simulink library "ada"  (Simulink 8.1)
settings: Solver=ode1  StartTime=0.0  StopTime=Inf  FixedStep=0.001  RelTol=1e-3
PostLoadFcn:
  | , if any(exist('dsrtsu_mdlpostloadfcn', 'file') == [2, 3, 6]), try dsrtsu_mdlpostloadfcn('Execute', bdroot); catch fprintf('Error in PostLoadFcn (dsrtsu_mdlpostloadfcn) for model "%s":\n %s\n', bdroot, lasterr); end, end,
settings Model: DSRTSU_INTERNAL_RTI_VER=450  DSRTSU_INTERNAL_RTI_TYPE=rti1401  RTICANMMDATA=struct('GeneralSetupData',struct('modelroot','D:\ELN150201\Phase3\trunk\Application\AdasDragon\software\sw_development\arch\app\ada','generalsettings',struct('filesettings',struct('destfolder',struct('Name','RTICANMM_FILES','Check',1),'buildfolder',struct('Name','.','Check',1),'AbsDestfolder',struct('Name','D:\ELN150201\Phase3\trunk\Application\AdasDragon\software\sw_development\arch\app\ada\RTICANMM_FILES'),'AbsBuildfolder',struct('Name','D:\ELN150201\Phase3\trunk\Application\AdasDragon\software\sw_development\arch\app\ada'))),'options',struct('addpaths',1,'rmpaths',1,'addtrcexclusion',logical(1),'cannavigator',struct('checkmonitoring',0),'show_usrtrc',0,'use_usrtrc',0),'advanced',struct('options',[1 1 1 1 1 1 1 1 1 1 1 1 1 1 1 1 1 1 1 1 1 1 1 1 1 1 1 1 1 1 1 1 1 1 1 1 1 1 1 1 1 1 1 1 1 1 1 1 1 1 1 1 1 1 1 1 1 1 1 1 1 1 1 1 1 1 1 1 1 1 1 1 1 1 1 1 1 1 1 1 1 1 1 1 1 1 1 1 1 1 1 1 1 1 1 1 1 1 1 1]),'MPSetup',{{}},'modelname','ada','block','ada'))  DSRTSU_INTERNAL_RTIFPGA=40  Creator=tescamilla  LastModifiedBy=AT015555

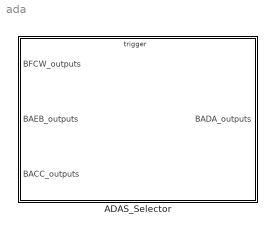
== system ada ==
  ADAS_Selector : Subsystem

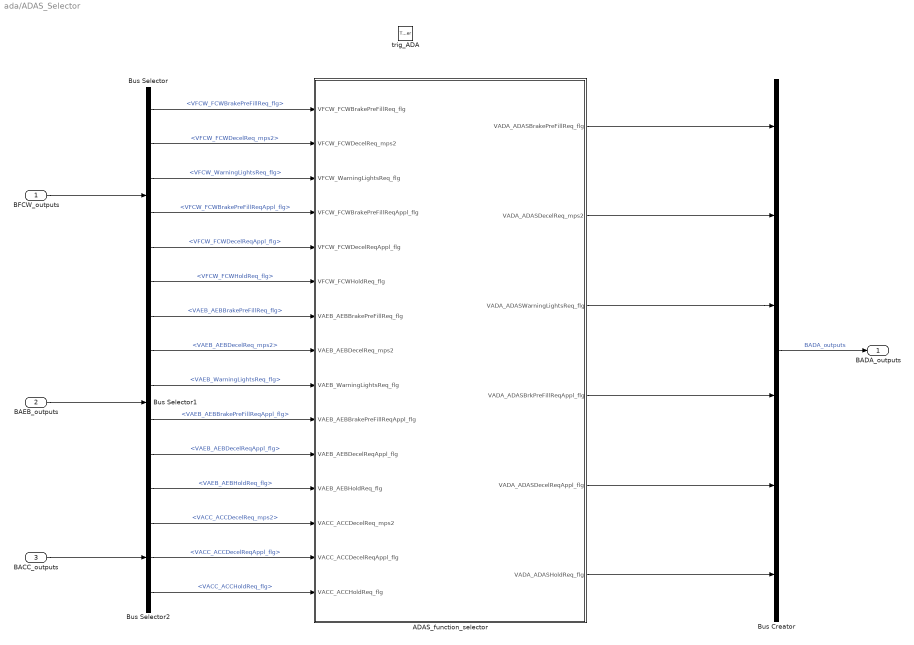
== system ada/ADAS_Selector ==
  BFCW_outputs : Inport  OutDataTypeStr=Bus: BFCW_outputs
  BAEB_outputs : Inport  Port=2  OutDataTypeStr=Bus: BAEB_outputs
  BACC_outputs : Inport  Port=3  OutDataTypeStr=Bus: BACC_outputs
  trig_ADA : TriggerPort  TriggerType=function-call
      settings: AttributesFormatString=State = %<StatesWhenEnabling>
  ADAS_function_selector : Subsystem
  Bus Creator : BusCreator  Inputs=6  OutDataTypeStr=Bus: BADA_outputs
  Bus Selector : BusSelector  OutputSignals=VFCW_FCWBrakePreFillReq_flg,VFCW_FCWDecelReq_mps2,VFCW_WarningLightsReq_flg,VFCW_FCWBrakePreFillReqAppl_flg,VFCW_FCWDecelReqAppl_flg,VFCW_FCWHoldReq_flg
  Bus Selector1 : BusSelector  OutputSignals=VAEB_AEBBrakePreFillReq_flg,VAEB_AEBDecelReq_mps2,VAEB_WarningLightsReq_flg,VAEB_AEBBrakePreFillReqAppl_flg,VAEB_AEBDecelReqAppl_flg,VAEB_AEBHoldReq_flg
  Bus Selector2 : BusSelector  OutputSignals=VACC_ACCDecelReq_mps2,VACC_ACCDecelReqAppl_flg,VACC_ACCHoldReq_flg
  BADA_outputs : Outport  OutDataTypeStr=Bus: BADA_outputs  LockScale=on
  wires:
  BFCW_outputs/1 -> Bus Selector/1
  BAEB_outputs/1 -> Bus Selector1/1
  Bus Selector1/5 -> ADAS_function_selector/11(VAEB_AEBDecelReqAppl_flg)  "<VAEB_AEBDecelReqAppl_flg>"
  Bus Selector1/1 -> ADAS_function_selector/7(VAEB_AEBBrakePreFillReq_flg)  "<VAEB_AEBBrakePreFillReq_flg>"
  Bus Selector/3 -> ADAS_function_selector/3(VFCW_WarningLightsReq_flg)  "<VFCW_WarningLightsReq_flg>"
  Bus Selector/6 -> ADAS_function_selector/6(VFCW_FCWHoldReq_flg)  "<VFCW_FCWHoldReq_flg>"
  Bus Selector/2 -> ADAS_function_selector/2(VFCW_FCWDecelReq_mps2)  "<VFCW_FCWDecelReq_mps2>"
  Bus Selector/5 -> ADAS_function_selector/5(VFCW_FCWDecelReqAppl_flg)  "<VFCW_FCWDecelReqAppl_flg>"
  Bus Selector/1 -> ADAS_function_selector/1(VFCW_FCWBrakePreFillReq_flg)  "<VFCW_FCWBrakePreFillReq_flg>"
  Bus Selector/4 -> ADAS_function_selector/4(VFCW_FCWBrakePreFillReqAppl_flg)  "<VFCW_FCWBrakePreFillReqAppl_flg>"
  Bus Selector1/3 -> ADAS_function_selector/9(VAEB_WarningLightsReq_flg)  "<VAEB_WarningLightsReq_flg>"
  Bus Selector1/2 -> ADAS_function_selector/8(VAEB_AEBDecelReq_mps2)  "<VAEB_AEBDecelReq_mps2>"
  Bus Selector1/4 -> ADAS_function_selector/10(VAEB_AEBBrakePreFillReqAppl_flg)  "<VAEB_AEBBrakePreFillReqAppl_flg>"
  Bus Selector1/6 -> ADAS_function_selector/12(VAEB_AEBHoldReq_flg)  "<VAEB_AEBHoldReq_flg>"
  ADAS_function_selector/1(VADA_ADASBrakePreFillReq_flg) -> Bus Creator/1
  Bus Creator/1 -> BADA_outputs/1  "BADA_outputs"
  ADAS_function_selector/3(VADA_ADASWarningLightsReq_flg) -> Bus Creator/3
  ADAS_function_selector/6(VADA_ADASHoldReq_flg) -> Bus Creator/6
  ADAS_function_selector/2(VADA_ADASDecelReq_mps2) -> Bus Creator/2
  ADAS_function_selector/5(VADA_ADASDecelReqAppl_flg) -> Bus Creator/5
  ADAS_function_selector/4(VADA_ADASBrkPreFillReqAppl_flg) -> Bus Creator/4
  BACC_outputs/1 -> Bus Selector2/1
  Bus Selector2/1 -> ADAS_function_selector/13(VACC_ACCDecelReq_mps2)  "<VACC_ACCDecelReq_mps2>"
  Bus Selector2/3 -> ADAS_function_selector/15(VACC_ACCHoldReq_flg)  "<VACC_ACCHoldReq_flg>"
  Bus Selector2/2 -> ADAS_function_selector/14(VACC_ACCDecelReqAppl_flg)  "<VACC_ACCDecelReqAppl_flg>"

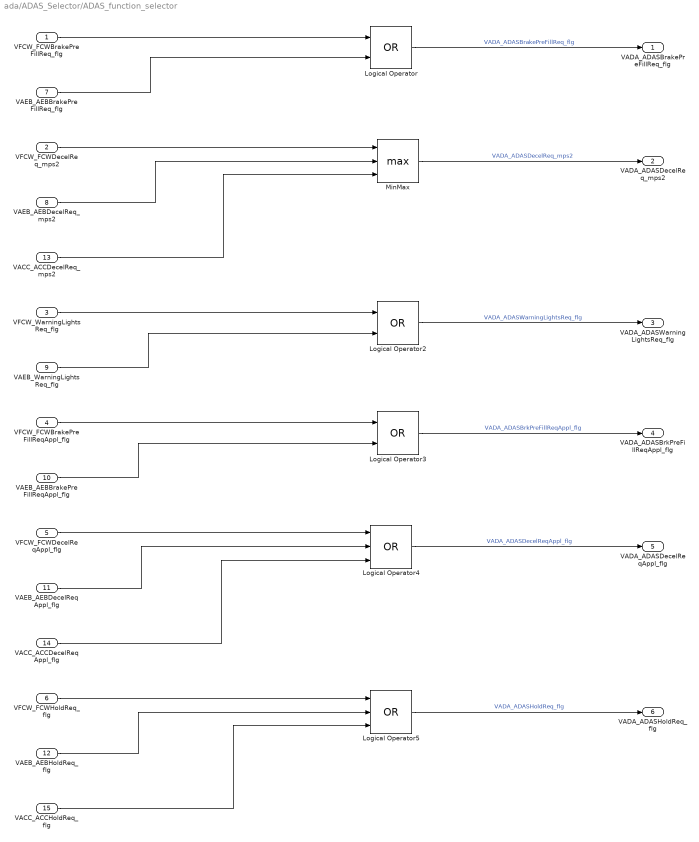
== system ada/ADAS_Selector/ADAS_function_selector ==
  VFCW_FCWBrakePreFillReq_flg : Inport
  VFCW_FCWDecelReq_mps2 : Inport  Port=2
  VFCW_WarningLightsReq_flg : Inport  Port=3
  VFCW_FCWBrakePreFillReqAppl_flg : Inport  Port=4
  VFCW_FCWDecelReqAppl_flg : Inport  Port=5
  VFCW_FCWHoldReq_flg : Inport  Port=6
  VAEB_AEBBrakePreFillReq_flg : Inport  Port=7
  VAEB_AEBDecelReq_mps2 : Inport  Port=8
  VAEB_WarningLightsReq_flg : Inport  Port=9
  VAEB_AEBBrakePreFillReqAppl_flg : Inport  Port=10
  VAEB_AEBDecelReqAppl_flg : Inport  Port=11
  VAEB_AEBHoldReq_flg : Inport  Port=12
  VACC_ACCDecelReq_mps2 : Inport  Port=13
  VACC_ACCDecelReqAppl_flg : Inport  Port=14
  VACC_ACCHoldReq_flg : Inport  Port=15
  Logical Operator : Logic  Operator=OR  AllPortsSameDT=off  OutDataTypeStr=boolean
  Logical Operator2 : Logic  Operator=OR  AllPortsSameDT=off  OutDataTypeStr=boolean
  Logical Operator3 : Logic  Operator=OR  AllPortsSameDT=off  OutDataTypeStr=boolean
  Logical Operator4 : Logic  Operator=OR  Inputs=3  AllPortsSameDT=off  OutDataTypeStr=boolean
  Logical Operator5 : Logic  Operator=OR  Inputs=3  AllPortsSameDT=off  OutDataTypeStr=boolean
  MinMax : MinMax  Function=max  Inputs=3
  VADA_ADASBrakePreFillReq_flg : Outport
  VADA_ADASDecelReq_mps2 : Outport  Port=2
  VADA_ADASWarningLightsReq_flg : Outport  Port=3
  VADA_ADASBrkPreFillReqAppl_flg : Outport  Port=4
  VADA_ADASDecelReqAppl_flg : Outport  Port=5
  VADA_ADASHoldReq_flg : Outport  Port=6
  wires:
  VFCW_FCWBrakePreFillReq_flg/1 -> Logical Operator/1
  VAEB_AEBBrakePreFillReq_flg/1 -> Logical Operator/2
  VFCW_FCWDecelReq_mps2/1 -> MinMax/1
  VAEB_AEBDecelReq_mps2/1 -> MinMax/2
  VFCW_WarningLightsReq_flg/1 -> Logical Operator2/1
  VAEB_WarningLightsReq_flg/1 -> Logical Operator2/2
  VFCW_FCWBrakePreFillReqAppl_flg/1 -> Logical Operator3/1
  VAEB_AEBBrakePreFillReqAppl_flg/1 -> Logical Operator3/2
  VFCW_FCWDecelReqAppl_flg/1 -> Logical Operator4/1
  VAEB_AEBDecelReqAppl_flg/1 -> Logical Operator4/2
  VFCW_FCWHoldReq_flg/1 -> Logical Operator5/1
  VAEB_AEBHoldReq_flg/1 -> Logical Operator5/2
  Logical Operator/1 -> VADA_ADASBrakePreFillReq_flg/1  "VADA_ADASBrakePreFillReq_flg"
  MinMax/1 -> VADA_ADASDecelReq_mps2/1  "VADA_ADASDecelReq_mps2"
  Logical Operator2/1 -> VADA_ADASWarningLightsReq_flg/1  "VADA_ADASWarningLightsReq_flg"
  Logical Operator3/1 -> VADA_ADASBrkPreFillReqAppl_flg/1  "VADA_ADASBrkPreFillReqAppl_flg"
  Logical Operator4/1 -> VADA_ADASDecelReqAppl_flg/1  "VADA_ADASDecelReqAppl_flg"
  Logical Operator5/1 -> VADA_ADASHoldReq_flg/1  "VADA_ADASHoldReq_flg"
  VACC_ACCDecelReq_mps2/1 -> MinMax/3
  VACC_ACCDecelReqAppl_flg/1 -> Logical Operator4/3
  VACC_ACCHoldReq_flg/1 -> Logical Operator5/3
